simulink model "SecRwRtStFwdBkwdCtrl"  (R2024b)
settings: Solver=FixedStepDiscrete  StartTime=0.0  StopTime=10.0  FixedStep=0.01  RelTol=1e-3
undefined symbols (not defined in the file or in its folder): KeSMSuMdMotFinshdTm_Val, KeSMSuMdRetryTm1_Val, KeSMSuModeReqDurgTm_Val
libraries: StCtrlLibBkRecln x1
settings Model: Creator=sn2xws  LastModifiedBy=sn55gm
settings Model: ModifiedHistory=|
  | 2024.10.14 V3.0.0 bitmask 更改为变量接口
  | 25.7.7 V3.13.0 Md61 Md62新增Retry口
  | 25.12.04 V3.14.0 MD12防夹退出机制
settings SolverCC: AlgebraicLoopSolver=TrustRegion
settings DataIOCC: SaveFormat=StructureWithTime  ReturnWorkspaceOutputs=off
settings OptimizationCC: DefaultParameterBehavior=Inlined  EnhancedBackFolding=on  PassReuseOutputArgsAs=Individual arguments  ZeroExternalMemoryAtStartup=off  ZeroInternalMemoryAtStartup=off  OptimizeBlockOrder=speed  DifferentSizesBufferReuse=on  OptimizationCustomize=off  EfficientTunableParamExpr=on
settings DebuggingCC: ParameterTunabilityLossMsg=error  UnconnectedInputMsg=warning  UnconnectedOutputMsg=warning  UnconnectedLineMsg=warning  ArithmeticOperatorsInVariantConditions=warning
settings ModelReferenceCC: EnableRefExpFcnMdlSchedulingChecks=on  ModelReferenceNumInstancesAllowed=Single
settings SFSimCC: MATLABDynamicMemAlloc=off  CustomCodeUndefinedFunction=UseInterfaceOnly
settings RTWCC: Description=AUTOSAR  SystemTargetFile=autosar.tlc  GenCodeOnly=on  TemplateMakefile=ert_default_tmf  GenerateReport=on  IncludeHyperlinkInReport=on  LaunchReport=on  DataTypeReplacement=CDataTypesFixedWidth  GenerateTraceInfo=on  GenerateTraceReport=on  GenerateTraceReportSl=on  GenerateTraceReportSf=on  GenerateTraceReportEml=on  GPUComputeCapability=3.5
settings CodeAppCC: ForceParamTrailComments=on  IgnoreCustomStorageClasses=off  OperatorAnnotations=on  SimulinkDataObjDesc=on  SFDataObjDesc=on  InsertBlockDesc=on
settings STFCustomTargetCC: TargetLangStandard=C99 (ISO)  MultiwordLength=256  ParMdlRefBuildCompliant=on  CompOptLevelCompliant=on  IncludeMdlTerminateFcn=off  CombineOutputUpdateFcns=on  SuppressErrorStatus=on  ERTCustomFileBanners=on  SupportNonFinite=off  SupportComplex=off  SupportContinuousTime=off  SupportNonInlinedSFcns=off  RemoveResetFunc=on  MATLABClassNameForMDSCustomization=Simulink.SoftwareTarget.ERTCustomization  AutosarCompliant=on  UseToolchainInfoCompliant=on  LookupTableObjectStructAxisOrder=2,1,3,4,...  LUTObjectStructOrderEvenSpacing=Size,Table,Breakpoints  SystemTargetFile=autosar.tlc
settings ERTTargetCC: TargetLangStandard=C99 (ISO)  ConcurrentExecutionCompliant=off  IncludeMdlTerminateFcn=off  SuppressErrorStatus=on  SupportNonFinite=off  SupportComplex=off  ModelStepFunctionPrototypeControlCompliant=off  CPPClassGenCompliant=off  AutosarCompliant=on  LookupTableObjectStructAxisOrder=2,1,3,4,...  LUTObjectStructOrderEvenSpacing=Size,Table,Breakpoints  ERTCustomFileTemplate=example_file_process.tlc  ERTFilePackagingFormat=Compact  BooleanTrueId=TRUE  BooleanFalseId=FALSE  DynamicArrayContainerType=coder::array

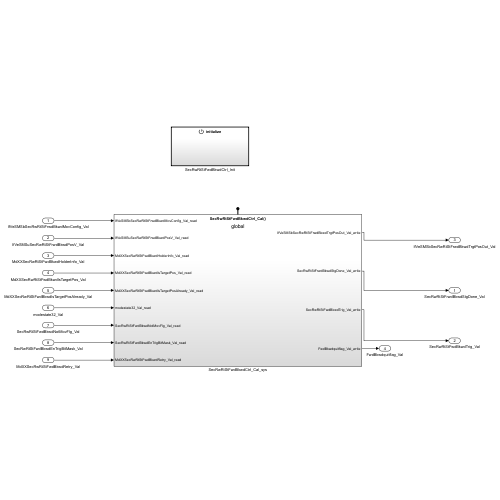
[thumbnail: Simulink's stored preview of the top-level diagram]
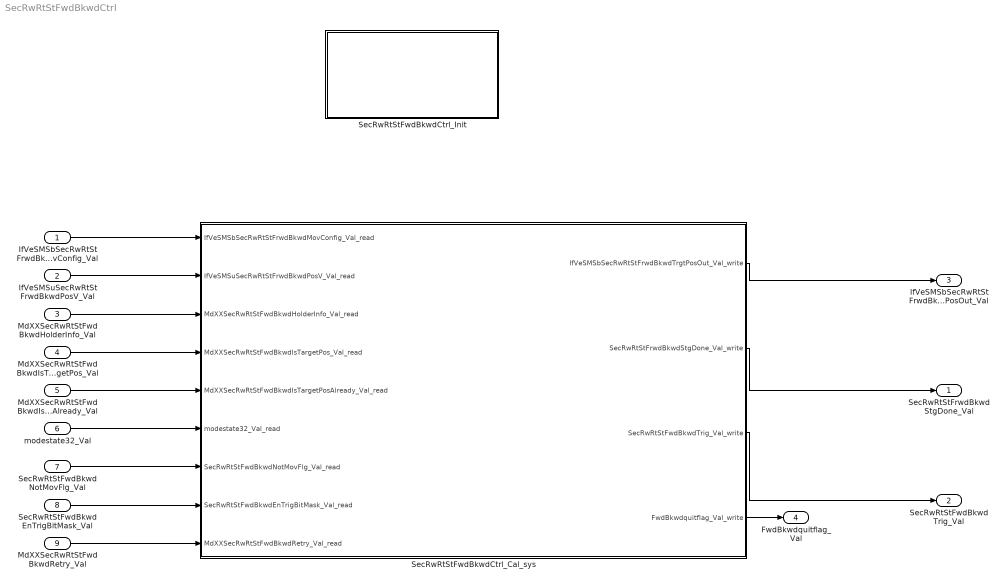
== system SecRwRtStFwdBkwdCtrl ==
  IfVeSMSbSecRwRtStFrwdBkwdMovConfig_Val : Inport  OutDataTypeStr=boolean  PortDimensions=1
  IfVeSMSuSecRwRtStFrwdBkwdPosV_Val : Inport  Port=2  OutDataTypeStr=boolean  PortDimensions=1
  MdXXSecRwRtStFwdBkwdHolderInfo_Val : Inport  Port=3  OutDataTypeStr=uint32  PortDimensions=1
  MdXXSecRwRtStFwdBkwdIsTargetPos_Val : Inport  Port=4  OutDataTypeStr=uint32  PortDimensions=1
  MdXXSecRwRtStFwdBkwdIsTargetPosAlready_Val : Inport  Port=5  OutDataTypeStr=uint32  PortDimensions=1
  modestate32_Val : Inport  Port=6  OutDataTypeStr=uint32  PortDimensions=1
  SecRwRtStFwdBkwdNotMovFlg_Val : Inport  Port=7  OutDataTypeStr=boolean  PortDimensions=1
  SecRwRtStFwdBkwdEnTrigBitMask_Val : Inport  Port=8  OutDataTypeStr=uint32  PortDimensions=1
  MdXXSecRwRtStFwdBkwdRetry_Val : Inport  Port=9  OutDataTypeStr=uint32  PortDimensions=1
  SecRwRtStFwdBkwdCtrl_Cal_sys : Subsystem
  SecRwRtStFwdBkwdCtrl_Init : Subsystem
  SecRwRtStFrwdBkwdStgDone_Val : Outport  OutDataTypeStr=boolean  PortDimensions=1  VectorParamsAs1DForOutWhenUnconnected=off
  SecRwRtStFwdBkwdTrig_Val : Outport  Port=2  OutDataTypeStr=boolean  PortDimensions=1  VectorParamsAs1DForOutWhenUnconnected=off
  IfVeSMSbSecRwRtStFrwdBkwdTrgtPosOut_Val : Outport  Port=3  OutDataTypeStr=boolean  PortDimensions=1  VectorParamsAs1DForOutWhenUnconnected=off
  FwdBkwdquitflag_Val : Outport  Port=4  OutDataTypeStr=boolean  PortDimensions=1  VectorParamsAs1DForOutWhenUnconnected=off
  wires:
  IfVeSMSbSecRwRtStFrwdBkwdMovConfig_Val/1 -> SecRwRtStFwdBkwdCtrl_Cal_sys/1(IfVeSMSbSecRwRtStFrwdBkwdMovConfig_Val_read)
  IfVeSMSuSecRwRtStFrwdBkwdPosV_Val/1 -> SecRwRtStFwdBkwdCtrl_Cal_sys/2(IfVeSMSuSecRwRtStFrwdBkwdPosV_Val_read)
  MdXXSecRwRtStFwdBkwdHolderInfo_Val/1 -> SecRwRtStFwdBkwdCtrl_Cal_sys/3(MdXXSecRwRtStFwdBkwdHolderInfo_Val_read)
  MdXXSecRwRtStFwdBkwdIsTargetPos_Val/1 -> SecRwRtStFwdBkwdCtrl_Cal_sys/4(MdXXSecRwRtStFwdBkwdIsTargetPos_Val_read)
  MdXXSecRwRtStFwdBkwdIsTargetPosAlready_Val/1 -> SecRwRtStFwdBkwdCtrl_Cal_sys/5(MdXXSecRwRtStFwdBkwdIsTargetPosAlready_Val_read)
  modestate32_Val/1 -> SecRwRtStFwdBkwdCtrl_Cal_sys/6(modestate32_Val_read)
  SecRwRtStFwdBkwdNotMovFlg_Val/1 -> SecRwRtStFwdBkwdCtrl_Cal_sys/7(SecRwRtStFwdBkwdNotMovFlg_Val_read)
  SecRwRtStFwdBkwdCtrl_Cal_sys/1(IfVeSMSbSecRwRtStFrwdBkwdTrgtPosOut_Val_write) -> IfVeSMSbSecRwRtStFrwdBkwdTrgtPosOut_Val/1
  SecRwRtStFwdBkwdCtrl_Cal_sys/2(SecRwRtStFrwdBkwdStgDone_Val_write) -> SecRwRtStFrwdBkwdStgDone_Val/1
  SecRwRtStFwdBkwdCtrl_Cal_sys/3(SecRwRtStFwdBkwdTrig_Val_write) -> SecRwRtStFwdBkwdTrig_Val/1
  SecRwRtStFwdBkwdEnTrigBitMask_Val/1 -> SecRwRtStFwdBkwdCtrl_Cal_sys/8(SecRwRtStFwdBkwdEnTrigBitMask_Val_read)
  MdXXSecRwRtStFwdBkwdRetry_Val/1 -> SecRwRtStFwdBkwdCtrl_Cal_sys/9(MdXXSecRwRtStFwdBkwdRetry_Val_read)
  SecRwRtStFwdBkwdCtrl_Cal_sys/4(FwdBkwdquitflag_Val_write) -> FwdBkwdquitflag_Val/1

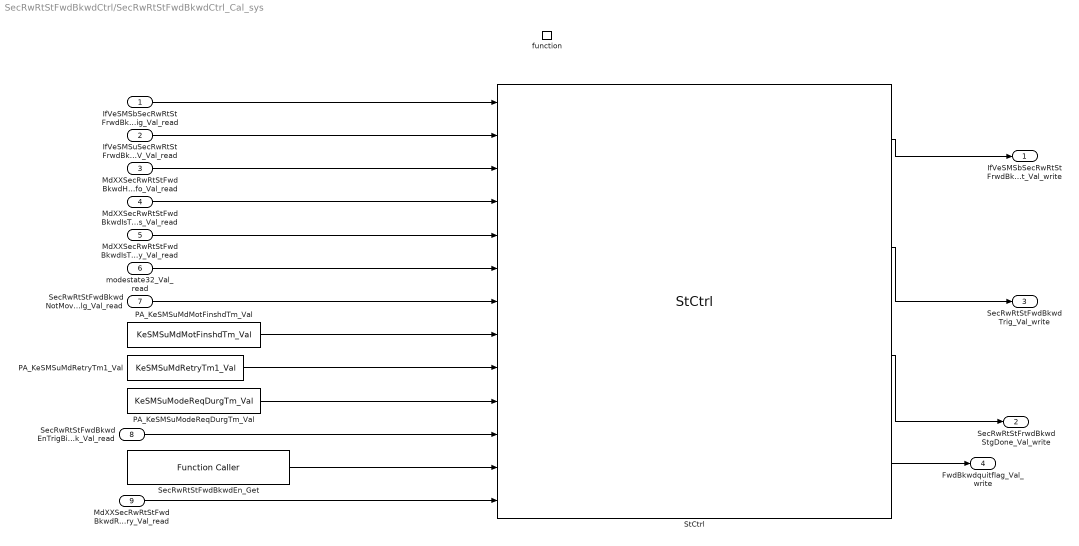
== system SecRwRtStFwdBkwdCtrl/SecRwRtStFwdBkwdCtrl_Cal_sys ==
  IfVeSMSbSecRwRtStFrwdBkwdMovConfig_Val_read : Inport
  IfVeSMSuSecRwRtStFrwdBkwdPosV_Val_read : Inport  Port=2
  MdXXSecRwRtStFwdBkwdHolderInfo_Val_read : Inport  Port=3
  MdXXSecRwRtStFwdBkwdIsTargetPos_Val_read : Inport  Port=4
  MdXXSecRwRtStFwdBkwdIsTargetPosAlready_Val_read : Inport  Port=5
  modestate32_Val_read : Inport  Port=6
  SecRwRtStFwdBkwdNotMovFlg_Val_read : Inport  Port=7
  SecRwRtStFwdBkwdEnTrigBitMask_Val_read : Inport  Port=8
  MdXXSecRwRtStFwdBkwdRetry_Val_read : Inport  Port=9
  function : TriggerPort  TriggerType=function-call  IsSimulinkFunction=on  FunctionName=SecRwRtStFwdBkwdCtrl_Cal  VariantControl=(inherit)
  PA_KeSMSuMdMotFinshdTm_Val : Constant  Value=KeSMSuMdMotFinshdTm_Val
  PA_KeSMSuMdRetryTm1_Val : Constant  Value=KeSMSuMdRetryTm1_Val
  PA_KeSMSuModeReqDurgTm_Val : Constant  Value=KeSMSuModeReqDurgTm_Val
  SecRwRtStFwdBkwdEn_Get : FunctionCaller  FunctionPrototype=data = SecRwRtStFwdBkwdEn_Get()  InputArgumentSpecifications=<Enter example>  OutputArgumentSpecifications=uint32(1)
  StCtrl : StCtrlLibBkRecln/StCtrl  SystemSampleTime=-1  VariantActivationTime=update diagram  AllowFlexibleInterface=on  Latency=0  AutoFrameSizeCalculation=off
  IfVeSMSbSecRwRtStFrwdBkwdTrgtPosOut_Val_write : Outport  VectorParamsAs1DForOutWhenUnconnected=off
      settings: EnsureOutportIsVirtual=on
  SecRwRtStFrwdBkwdStgDone_Val_write : Outport  Port=2  VectorParamsAs1DForOutWhenUnconnected=off
      settings: EnsureOutportIsVirtual=on
  SecRwRtStFwdBkwdTrig_Val_write : Outport  Port=3  VectorParamsAs1DForOutWhenUnconnected=off
      settings: EnsureOutportIsVirtual=on
  FwdBkwdquitflag_Val_write : Outport  Port=4  VectorParamsAs1DForOutWhenUnconnected=off
      settings: EnsureOutportIsVirtual=on
  wires:
  SecRwRtStFwdBkwdEnTrigBitMask_Val_read/1 -> StCtrl/11
  SecRwRtStFwdBkwdEn_Get/1 -> StCtrl/12
  PA_KeSMSuMdMotFinshdTm_Val/1 -> StCtrl/8
  PA_KeSMSuModeReqDurgTm_Val/1 -> StCtrl/10
  PA_KeSMSuMdRetryTm1_Val/1 -> StCtrl/9
  IfVeSMSbSecRwRtStFrwdBkwdMovConfig_Val_read/1 -> StCtrl/1
  IfVeSMSuSecRwRtStFrwdBkwdPosV_Val_read/1 -> StCtrl/2
  MdXXSecRwRtStFwdBkwdHolderInfo_Val_read/1 -> StCtrl/3
  MdXXSecRwRtStFwdBkwdIsTargetPos_Val_read/1 -> StCtrl/4
  MdXXSecRwRtStFwdBkwdIsTargetPosAlready_Val_read/1 -> StCtrl/5
  modestate32_Val_read/1 -> StCtrl/6
  SecRwRtStFwdBkwdNotMovFlg_Val_read/1 -> StCtrl/7
  StCtrl/1 -> IfVeSMSbSecRwRtStFrwdBkwdTrgtPosOut_Val_write/1
  StCtrl/2 -> SecRwRtStFwdBkwdTrig_Val_write/1
  StCtrl/3 -> SecRwRtStFrwdBkwdStgDone_Val_write/1
  MdXXSecRwRtStFwdBkwdRetry_Val_read/1 -> StCtrl/13
  StCtrl/4 -> FwdBkwdquitflag_Val_write/1

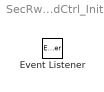
== system SecRwRtStFwdBkwdCtrl/SecRwRtStFwdBkwdCtrl_Init ==
  Event Listener : EventListener  EventName=reset
